simulink model "fixed_model"  (R2024a)
settings: Solver=VariableStepAuto  StartTime=0.0  StopTime=1  RelTol=1e-3
values from neighbouring files (symbols this model uses):
  SAMPLING_FREQ = 12800    [workspace.mat]
  signal_1 = [0 0.0001 0.0002 0.0003 0.0004 0.0005 0.0006 0.0007 0.0008 0.0009 0.001 0.0011 ... (4096 elements, 2048x2)]    [workspace.mat]
libraries: dspstat3 x3, dspsrcs4 x1, dspxfrm3 x1, simulink x1
settings Model: FPTShortcutValueString='{{},{''BaselineRun_3'',1,1,1,''BaselineRun_3'','''',{},''M'',''D'',''''},{''BaselineRun'',1,1,1,''BaselineRun'','''',{},''M'',''D'',''''}}'  SimulationMode=accelerator  Creator=Jan Rosa  LastModifiedBy=Jan Rosa
settings DebuggingCC: SignalRangeChecking=warning
settings HardwareCC: ProdBitPerPointer=32  ProdBitPerSizeT=32  ProdBitPerPtrDiffT=32  ProdLargestAtomicFloat=None  ProdIntDivRoundTo=Undefined  ProdEndianess=Unspecified  ProdWordSize=32  ProdHWDeviceType=ASIC/FPGA->ASIC/FPGA  TargetBitPerPointer=64  TargetBitPerSizeT=64  TargetBitPerPtrDiffT=64  TargetLongLongMode=on  TargetIntDivRoundTo=Zero  TargetEndianess=LittleEndian  TargetWordSize=64  TargetHWDeviceType=Custom Processor->MATLAB Host Computer  ProdEqTarget=off

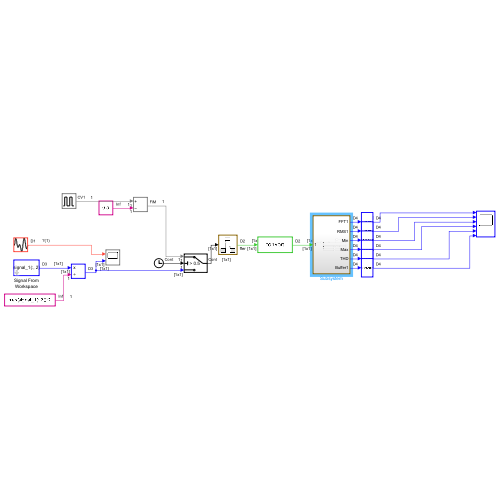
[thumbnail: Simulink's stored preview of the top-level diagram]
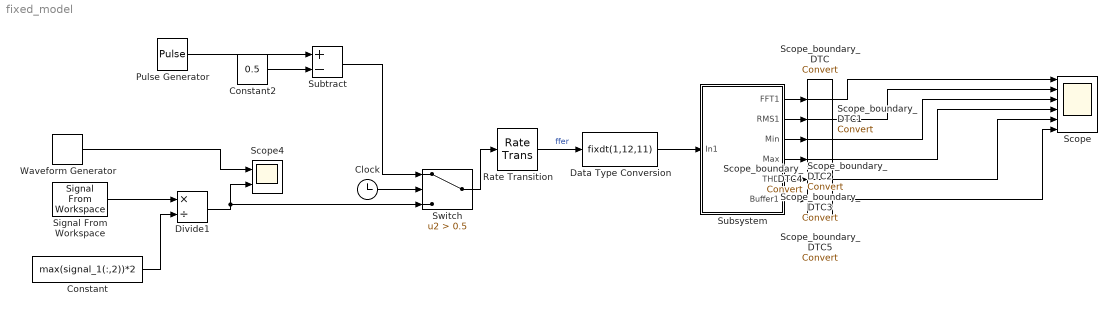
== system fixed_model ==
  Clock : Clock
  Constant : Constant  Value=max(signal_1(:,2))*2
  Constant2 : Constant  Value=0.5
  Data Type Conversion : DataTypeConversion  OutDataTypeStr=fixdt(1,12,11)  SaturateOnIntegerOverflow=off  RndMeth=Floor
  Divide1 : Product  Inputs=*/
  Pulse Generator : DiscretePulseGenerator  PulseType=Time based  Amplitude=0.999  Period=1/50  PulseWidth=50
  Rate Transition : RateTransition  Deterministic=off  OutPortSampleTime=1/SAMPLING_FREQ
  Scope : Scope  NumInputPorts=6
  Scope4 : Scope  NumInputPorts=2
  Scope_boundary_DTC{,1..5} (6 alike) : DataTypeConversion
  Signal From Workspace : dspsrcs4/Signal From Workspace  X=signal_1(:, 2)  Ts=signal_1(2, 1)  nsamps=1  OutputAfterFinalValue=Cyclic repetition  ignoreOrWarnInputAndFrameLengths=off  OutputFrames=off
  Subsystem : Subsystem
  Subtract : Sum  Inputs=+-
  Switch : Switch  Criteria=u2 > Threshold  Threshold=0.5  SaturateOnIntegerOverflow=off  InputSameDT=off
  Waveform Generator : simulink/Sources/Waveform Generator  OutMin=[]  OutMax=[]  OutDataTypeStr=double  SelectedSignal=1  Signals=0.99*sin(0.5, 50*2*pi, 0)  BlockNames=MultiportSwitch_c7ceefe4d1e8441  SampleTime=1/(SAMPLING_FREQ*2)
  wires:
  Rate Transition/1 -> Data Type Conversion/1  "ffer"
  Signal From Workspace/1 -> Divide1/1
  Constant/1 -> Divide1/2
  Waveform Generator/1 -> Scope4/1
  Divide1/1 -> Switch/3, Scope4/2
  Pulse Generator/1 -> Subtract/1
  Constant2/1 -> Subtract/2
  Data Type Conversion/1 -> Subsystem/1(In1)
  Clock/1 -> Switch/2
  Subtract/1 -> Switch/1
  Switch/1 -> Rate Transition/1
  Subsystem/1(FFT1) -> Scope_boundary_DTC/1
  Scope_boundary_DTC/1 -> Scope/1
  Subsystem/2(RMS1) -> Scope_boundary_DTC1/1
  Scope_boundary_DTC1/1 -> Scope/2
  Subsystem/3(Min) -> Scope_boundary_DTC2/1
  Scope_boundary_DTC2/1 -> Scope/3
  Subsystem/4(Max) -> Scope_boundary_DTC3/1
  Scope_boundary_DTC3/1 -> Scope/4
  Subsystem/5(THD) -> Scope_boundary_DTC4/1
  Scope_boundary_DTC4/1 -> Scope/5
  Subsystem/6(Buffer1) -> Scope_boundary_DTC5/1
  Scope_boundary_DTC5/1 -> Scope/6

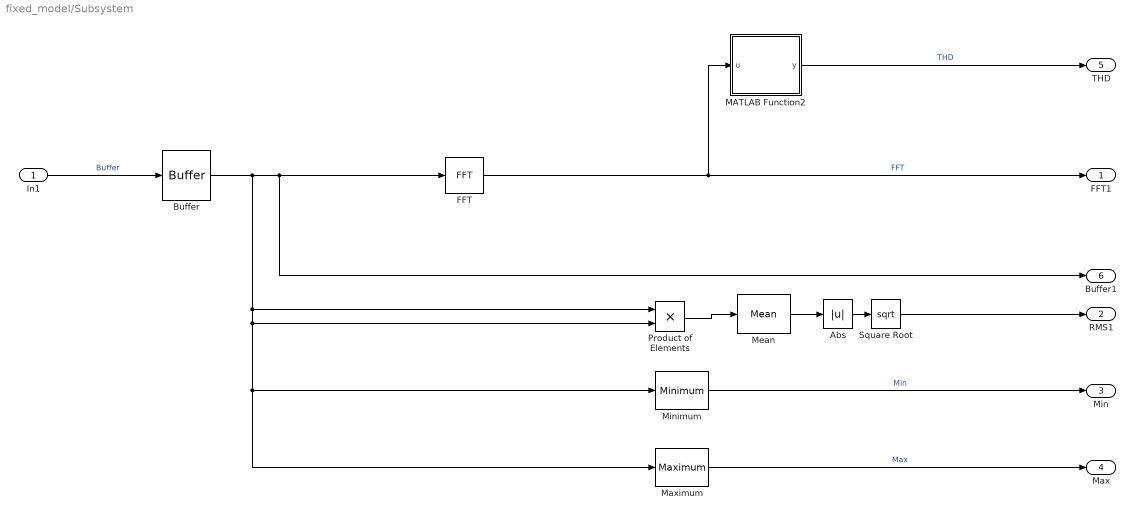
== system fixed_model/Subsystem ==
  In1 : Inport  OutDataTypeStr=fixdt(1,12,11)
  Abs : Abs  OutDataTypeStr=fixdt(0,12,11)  SaturateOnIntegerOverflow=off
  Buffer : Buffer  N=2048  V=2047  OutputFrames=off
  FFT : dspxfrm3/FFT  FFTImplementation=Auto  CompMethod=Table lookup  TableOpt=NEW  TableOptActive=Speed  BitRevOrder=off  Normalize=off  InheritFFTLength=on  FFTLength=64  WrapInput=on  roundingMode=Ceiling  overflowMode=off  firstCoeffDataTypeStr=Inherit: Same word length as input  firstCoeffLastDataTypeStr=Inherit: Same word length as input  outputMin=[]  outputMax=[]
  MATLAB Function2 : Subsystem  TreatAsAtomicUnit=on  Variant=on  VariantControlMode=label  VariantControl=MATLAB Function2  LabelModeActiveChoice=false()
  Maximum : dspstat3/Maximum  operation=maximum  fcn=Value  indexBase=One  operateOver=Each column  Dimension=1  InputProcessing=Columns as channels (frame based)  reset=None  roiEnable=off  roiType=Rectangles  roiPortion=Entire ROI  roiOutput=Individual statistics for each ROI  roiFlag=off  roundingMode=Floor  overflowMode=off  accumDataTypeStr=Inherit: Same as product output  accumLastDataTypeStr=Inherit: Same as product output
  Mean : dspstat3/Mean  run=off  InputProcessing=Columns as channels (frame based)  reset_popup=None  directionMode=Each column  dimension=1  roiEnable=off  roiType=Rectangles  roiPortion=Entire ROI  roiOutput=Individual statistics for each ROI  roiFlag=off  roundingMode=Floor  overflowMode=off  accumMode=Binary point scaling  accumWordLength=22  accumFracLength=11  accumDataTypeStr=fixdt([],22,11)  accumLastDataTypeStr=fixdt([],22,11)  outputMode=Binary point scaling  outputWordLength=12  outputFracLength=11  outputDataTypeStr=fixdt([],12,11)  outputMin=[]  outputMax=[]  outputLastDataTypeStr=fixdt([],12,11)
  Minimum : dspstat3/Minimum  operation=minimum  fcn=Value  indexBase=One  operateOver=Entire input  Dimension=1  InputProcessing=Columns as channels (frame based)  reset=None  roiEnable=off  roiType=Rectangles  roiPortion=Entire ROI  roiOutput=Individual statistics for each ROI  roiFlag=off  roundingMode=Floor  overflowMode=off
      settings: LibrarySourceBlock=dsphdlsupportstat/Minimum
  Product of Elements : Product  Inputs=**
  Square Root : Sqrt  OutDataTypeStr=fixdt(1,12,11)
  FFT1 : Outport
  RMS1 : Outport  Port=2
  Min : Outport  Port=3
  Max : Outport  Port=4
  THD : Outport  Port=5
  Buffer1 : Outport  Port=6
  wires:
  FFT/1 -> FFT1/1, MATLAB Function2/1(u)  "FFT"
  In1/1 -> Buffer/1  "Buffer"
  Minimum/1 -> Min/1  "Min"
  Maximum/1 -> Max/1  "Max"
  Product of Elements/1 -> Mean/1
  Mean/1 -> Abs/1
  Square Root/1 -> RMS1/1
  MATLAB Function2/1(y) -> THD/1  "THD"
  Abs/1 -> Square Root/1
  Buffer/1 -> FFT/1, Buffer1/1, Product of Elements/1, Product of Elements/2, Minimum/1, Maximum/1

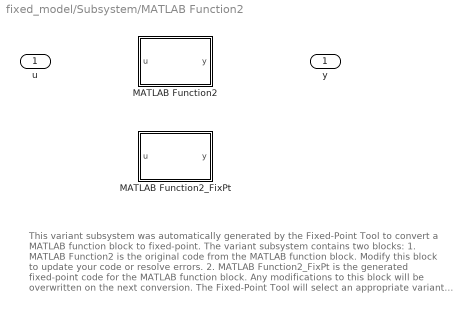
== system fixed_model/Subsystem/MATLAB Function2 ==
  note: This variant subsystem was automatically generated by the Fixed-Point Tool to convert a MATLAB function block to fixed-point.
      |
      | The variant subsystem contains two blocks:
      | 1. MATLAB Function2 is the original code from the MATLAB function block. Modify this block to update your code or resolve errors.
      |
      | 2. MATLAB Function2_FixPt is the generated fixed-point code for the MATLAB function block. Any modifications to this block will be overwritten on the next conversion.
      |
      | The Fixed-Point Tool will select an appropriate variant based on the Model Settings. Learn more.
  u : Inport
  MATLAB Function2 : MATLAB Function  TreatAsAtomicUnit=on  VariantControl=false()
  MATLAB Function2_FixPt : MATLAB Function  TreatAsAtomicUnit=on  VariantControl=(default)
  y : Outport

== matlab function fixed_model/Subsystem/MATLAB Function2/MATLAB Function2 ==
  data: u input; y output
function y = myTHD(u)

    u_abs = abs(u);
    main_frequency_index = 9;
    main_frequency_abs = u_abs(main_frequency_index);
    halfway_index = 1024;
    u_abs_square = u_abs(main_frequency_index+1:halfway_index).^2;
    u_abs_SM = sum(u_abs_square);
    
y = (sqrt(u_abs_SM))/main_frequency_abs;

== matlab function fixed_model/Subsystem/MATLAB Function2/MATLAB Function2_FixPt ==
  settings: fimath=fimath('RoundingMethod', 'Floor', 'OverflowAction', 'Wrap', 'ProductMode', 'FullPrecision', 'MaxProductWordLength', 128, 'SumMode', 'FullPrecision', 'MaxSumWordLength', 128)
  data: u input; y output
%auto-generated
%#codegen
function y = myTHD_fixpt(u)

    fm = get_fimath();
    u = fi(u, 1, 16, 15, fm);

    u_abs = fi(abs(u), 0, 16, 17, fm);
    main_frequency_index = fi(9, 0, 16, 12, fm);
    main_frequency_abs = fi(u_abs(main_frequency_index), 0, 16, 17, fm);
    halfway_index = fi(1024, 0, 16, 5, fm);
    u_abs_square = fi(u_abs(main_frequency_index+fi(1, 0, 1, 0, fm):halfway_index).^2, 0, 16, 20, fm);
    u_abs_SM = fi(sum(u_abs_square), 0, 16, 20, fm);
    
y = fi(fi_div((sqrt(u_abs_SM)), main_frequency_abs), 0, 16, 10, fm);
end



function ntype = divideType(a,b)
    coder.inline( 'always' );
    nt1 = numerictype( a );
    nt2 = numerictype( b );
    maxFL = max( [ min( nt1.WordLength, nt1.FractionLength ), min( nt2.WordLength, nt2.FractionLength ) ] );
    FL = max( maxFL, 24 );
    extraBits = (FL - maxFL);
    WL = nt1.WordLength + nt2.WordLength;
    WL = min( WL, 124 );
    if (WL + extraBits)<64
        ntype = numerictype( nt1.Signed || nt2.Signed, WL + extraBits, FL );
    else
        ntype = numerictype( nt1.Signed || nt2.Signed, WL, FL );
    end
end


function c = fi_div(a,b)
    coder.inline( 'always' );
    a1 = fi( a, 'RoundMode', 'fix' );
    b1 = fi( b, 'RoundMode', 'fix' );
    nType = divideType( a1, b1 );
    if isfi( a ) && isfi( b ) && isscalar( b )
        c1 = divide( nType, a1, b1 );
        c = fi( c1, numerictype( c1 ), fimath( a ) );
    else
        c = fi( a / b, nType );
    end
end

function fm = get_fimath()
	fm = fimath('RoundingMethod', 'Floor',...
	     'OverflowAction', 'Wrap',...
	     'ProductMode','FullPrecision',...
	     'MaxProductWordLength', 128,...
	     'SumMode','FullPrecision',...
	     'MaxSumWordLength', 128);
end
